simulink model "ControlPendulo2GDL_CICD"  (R2019b)
settings: Solver=ode4  StartTime=0.0  StopTime=ts  FixedStep=0.01  RelTol=1e-3
values from neighbouring files (symbols this model uses):
  b1 = c8    (= 0.01)    [PenduloDatos.m]
  b2 = c8    (= 0.01)    [PenduloDatos.m]
  C = [1 0 0 0]    [PenduloDatos.m]
  g = 9.78    [PenduloDatos.m]
  I1 = 1/12*m1*(a1^2+d1^2)    (= 3.14166666667e-05)    [PenduloDatos.m]
  I2 = 1/12*m2*(a2^2+d2^2)    (= 1.20833333333e-05)    [PenduloDatos.m]
  K = place(Al,Bl,[Pd1 Pd2 Pd3 Pd4])    [PenduloDatos.m]
  K0 = inv(C*(inv(-Al+Bl*K))*Bl)    [PenduloDatos.m]
  L = place(Al',C',[5*Pd1 5*Pd2 5*Pd3 5*Pd4])'    [PenduloDatos.m]
  l1 = c1    (= 0.3)    [PenduloDatos.m]
  l2 = c2    (= 0.2)    [PenduloDatos.m]
  lc1 = 0.25    [PenduloDatos.m]
  lc2 = 0.11    [PenduloDatos.m]
  m1 = c3    (= 0.065)    [PenduloDatos.m]
  m2 = c4    (= 0.025)    [PenduloDatos.m]
  U0 = [Tau1]    [PenduloDatos.m]
  X0 = [Tt1;Tpt1;Tt2;Tpt2]    [PenduloDatos.m]
  XI = [0;0;0;0]    [PenduloDatos.m]
undefined symbols (not defined in the file or in its folder): Al, Bl
libraries: simulink x4
settings Model: Creator=ARQ SEVILLA R  LastModifiedBy=ARQ SEVILLA R

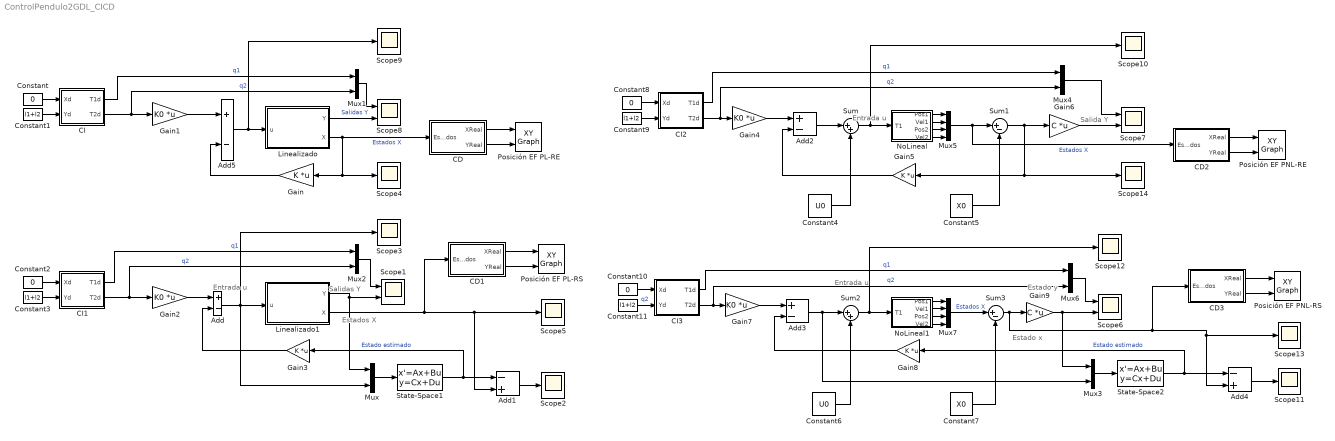
== system ControlPendulo2GDL_CICD ==
  note: Estados X
  note: Salidas Y
  note: Entrada u
  note: Salida Y
  note: Entrada u
  note: Entrada u
  note: Estado y
  note: Estado x
  Add{,2..3,5} (4 alike) : Sum  Inputs=+-
  Add1 : Sum  Inputs=-+
  Add4 : Sum  Inputs=-+
  CD : Subsystem  TreatAsAtomicUnit=on
  CD1 : Subsystem  TreatAsAtomicUnit=on
  CD2 : Subsystem  TreatAsAtomicUnit=on
  CD3 : Subsystem  TreatAsAtomicUnit=on
  CI : Subsystem  TreatAsAtomicUnit=on
  CI1 : Subsystem  TreatAsAtomicUnit=on
  CI2 : Subsystem  TreatAsAtomicUnit=on
  CI3 : Subsystem  TreatAsAtomicUnit=on
  Constant{,2,8,10} (4 alike) : Constant  Value=0
  Constant{1,3,9,11} (4 alike) : Constant  Value=l1+l2
  Constant4 : Constant  Value=U0
  Constant5 : Constant  Value=X0
  Constant6 : Constant  Value=U0
  Constant7 : Constant  Value=X0
  Gain{,3,5,8} (4 alike) : Gain  Gain=K  Multiplication=Matrix(K*u)
  Gain{1..2,4,7} (4 alike) : Gain  Gain=K0  Multiplication=Matrix(K*u)
  Gain6 : Gain  Gain=C  Multiplication=Matrix(K*u)
  Gain9 : Gain  Gain=C  Multiplication=Matrix(K*u)
  Linealizado : Subsystem
  Linealizado1 : Subsystem
  Mux{,1..4,6} (6 alike) : Mux  Inputs=2
  Mux5 : Mux
  Mux7 : Mux
  NoLineal : Subsystem
  NoLineal1 : Subsystem
  Posición EF PL-RE : simulink/Sinks/XY Graph  xmin=-l2-l1  xmax=l2+l1  ymin=-l2-l1  ymax=l2+l1  st=-1
  Posición EF PL-RS : simulink/Sinks/XY Graph  xmin=-l2-l1  xmax=l2+l1  ymin=-l2-l1  ymax=l2+l1  st=-1
  Posición EF PNL-RE : simulink/Sinks/XY Graph  xmin=-l2-l1  xmax=l2+l1  ymin=-l2-l1  ymax=l2+l1  st=-1
  Posición EF PNL-RS : simulink/Sinks/XY Graph  xmin=-l2-l1  xmax=l2+l1  ymin=-l2-l1  ymax=l2+l1  st=-1
  Scope{1,6..8} (4 alike) : Scope  NumInputPorts=2
  Scope{2..5,9..14} (10 alike) : Scope
  State-Space1 : StateSpace  A=Al-L*C  B=[L,Bl]  C=eye(4)  D=zeros(4,2)  InitialCondition=XI
  State-Space2 : StateSpace  A=Al-L*C  B=[L,Bl]  C=eye(4)  D=zeros(4,2)  InitialCondition=XI
  Sum : Sum  Inputs=|++
  Sum1 : Sum  Inputs=|+-
  Sum2 : Sum  Inputs=|++
  Sum3 : Sum  Inputs=|+-
  wires:
  CI/1(T1d) -> Mux1/1  "q1"
  Linealizado/2(X) -> CD/1(Estados), Scope4/1, Gain/1  "Estados X"
  Add5/1 -> Scope9/1, Linealizado/1(u)
  Gain1/1 -> Add5/1
  Linealizado1/2(X) -> CD1/1(Estados), Scope5/1, Add1/2
  Add/1 -> Linealizado1/1(u), Mux/2, Scope3/1
  Gain2/1 -> Add/1
  Linealizado1/1(Y) -> Scope1/2, Mux/1
  Mux/1 -> State-Space1/1
  Add1/1 -> Scope2/1
  Gain3/1 -> Add/2
  State-Space1/1 -> Add1/1, Gain3/1  "Estado estimado"
  CD/1(XReal) -> Posición EF PL-RE/1
  CD/2(YReal) -> Posición EF PL-RE/2
  Constant/1 -> CI/1(Xd)
  Constant1/1 -> CI/2(Yd)
  CI/2(T2d) -> Gain1/1, Mux1/2  "q2"
  Mux1/1 -> Scope8/1
  Linealizado/1(Y) -> Scope8/2  "Salidas Y"
  Gain/1 -> Add5/2
  CD1/2(YReal) -> Posición EF PL-RS/2
  CD1/1(XReal) -> Posición EF PL-RS/1
  Constant2/1 -> CI1/1(Xd)
  Mux2/1 -> Scope1/1
  CI1/1(T1d) -> Mux2/1  "q1"
  Add2/1 -> Sum/1
  Sum/1 -> Scope10/1, NoLineal/1(T1)
  Sum1/1 -> Scope14/1, Gain5/1, Gain6/1
  Sum2/1 -> NoLineal1/1(T1), Scope12/1
  Constant5/1 -> Sum1/2
  Add4/1 -> Scope11/1
  Constant4/1 -> Sum/2
  State-Space2/1 -> Add4/1, Gain8/1  "Estado estimado"
  Constant7/1 -> Sum3/2
  Sum3/1 -> CD3/1(Estados), Scope13/1, Add4/2, Gain9/1
  Add3/1 -> Mux3/2, Sum2/1
  Gain7/1 -> Add3/1
  Gain8/1 -> Add3/2
  Constant6/1 -> Sum2/2
  Gain9/1 -> Mux3/1, Scope6/2
  Gain4/1 -> Add2/1
  Mux3/1 -> State-Space2/1
  Gain5/1 -> Add2/2
  Gain6/1 -> Scope7/2
  Constant8/1 -> CI2/1(Xd)
  CI2/1(T1d) -> Mux4/1  "q1"
  Mux4/1 -> Scope7/1
  NoLineal/3(Pos2) -> Mux5/3
  Mux5/1 -> CD2/1(Estados), Sum1/1  "Estados X"
  NoLineal/4(Vel2) -> Mux5/4
  NoLineal/2(Vel1) -> Mux5/2
  NoLineal/1(Pos1) -> Mux5/1
  CD2/2(YReal) -> Posición EF PNL-RE/2
  CD2/1(XReal) -> Posición EF PNL-RE/1
  Constant10/1 -> CI3/1(Xd)
  Mux6/1 -> Scope6/1
  CI3/1(T1d) -> Mux6/1  "q1"
  CD3/1(XReal) -> Posición EF PNL-RS/1
  CD3/2(YReal) -> Posición EF PNL-RS/2
  NoLineal1/4(Vel2) -> Mux7/4
  NoLineal1/3(Pos2) -> Mux7/3
  NoLineal1/1(Pos1) -> Mux7/1
  NoLineal1/2(Vel1) -> Mux7/2
  Mux7/1 -> Sum3/1  "Estados X"
  Constant3/1 -> CI1/2(Yd)
  CI1/2(T2d) -> Mux2/2, Gain2/1  "q2"
  Constant9/1 -> CI2/2(Yd)
  CI2/2(T2d) -> Mux4/2, Gain4/1  "q2"
  Constant11/1 -> CI3/2(Yd)  "q2"
  CI3/2(T2d) -> Mux6/2, Gain7/1  "q2"

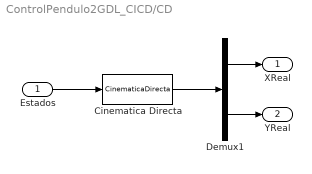
== system ControlPendulo2GDL_CICD/CD ==
  Estados : Inport
  Cinematica Directa : MATLABFcn  MATLABFcn=CinematicaDirecta  OutputDimensions=2
  Demux1 : Demux  Outputs=2
  XReal : Outport  VectorParamsAs1DForOutWhenUnconnected=off
  YReal : Outport  Port=2  VectorParamsAs1DForOutWhenUnconnected=off
  wires:
  Cinematica Directa/1 -> Demux1/1
  Demux1/1 -> XReal/1
  Demux1/2 -> YReal/1
  Estados/1 -> Cinematica Directa/1

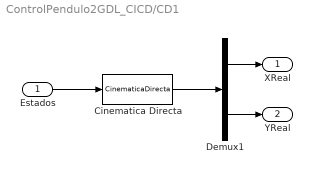
== system ControlPendulo2GDL_CICD/CD1 ==
  Estados : Inport
  Cinematica Directa : MATLABFcn  MATLABFcn=CinematicaDirecta  OutputDimensions=2
  Demux1 : Demux  Outputs=2
  XReal : Outport  VectorParamsAs1DForOutWhenUnconnected=off
  YReal : Outport  Port=2  VectorParamsAs1DForOutWhenUnconnected=off
  wires:
  Estados/1 -> Cinematica Directa/1
  Demux1/2 -> YReal/1
  Demux1/1 -> XReal/1
  Cinematica Directa/1 -> Demux1/1

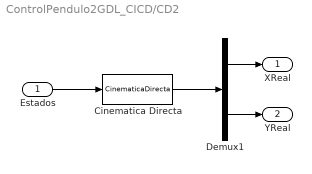
== system ControlPendulo2GDL_CICD/CD2 ==
  Estados : Inport
  Cinematica Directa : MATLABFcn  MATLABFcn=CinematicaDirecta  OutputDimensions=2
  Demux1 : Demux  Outputs=2
  XReal : Outport  VectorParamsAs1DForOutWhenUnconnected=off
  YReal : Outport  Port=2  VectorParamsAs1DForOutWhenUnconnected=off
  wires:
  Cinematica Directa/1 -> Demux1/1
  Demux1/1 -> XReal/1
  Demux1/2 -> YReal/1
  Estados/1 -> Cinematica Directa/1

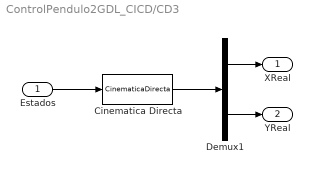
== system ControlPendulo2GDL_CICD/CD3 ==
  Estados : Inport
  Cinematica Directa : MATLABFcn  MATLABFcn=CinematicaDirecta  OutputDimensions=2
  Demux1 : Demux  Outputs=2
  XReal : Outport  VectorParamsAs1DForOutWhenUnconnected=off
  YReal : Outport  Port=2  VectorParamsAs1DForOutWhenUnconnected=off
  wires:
  Estados/1 -> Cinematica Directa/1
  Demux1/2 -> YReal/1
  Demux1/1 -> XReal/1
  Cinematica Directa/1 -> Demux1/1

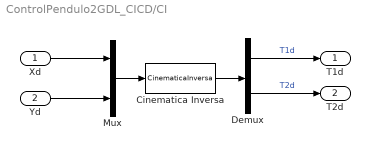
== system ControlPendulo2GDL_CICD/CI ==
  Xd : Inport
  Yd : Inport  Port=2
  Cinematica Inversa : MATLABFcn  MATLABFcn=CinematicaInversa  OutputDimensions=2
  Demux : Demux  Outputs=2
  Mux : Mux  Inputs=2
  T1d : Outport  VectorParamsAs1DForOutWhenUnconnected=off
  T2d : Outport  Port=2  VectorParamsAs1DForOutWhenUnconnected=off
  wires:
  Demux/2 -> T2d/1  "T2d"
  Demux/1 -> T1d/1  "T1d"
  Cinematica Inversa/1 -> Demux/1
  Mux/1 -> Cinematica Inversa/1
  Xd/1 -> Mux/1
  Yd/1 -> Mux/2

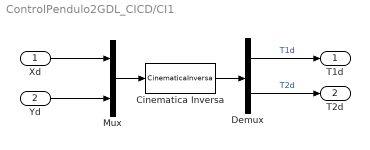
== system ControlPendulo2GDL_CICD/CI1 ==
  Xd : Inport
  Yd : Inport  Port=2
  Cinematica Inversa : MATLABFcn  MATLABFcn=CinematicaInversa  OutputDimensions=2
  Demux : Demux  Outputs=2
  Mux : Mux  Inputs=2
  T1d : Outport  VectorParamsAs1DForOutWhenUnconnected=off
  T2d : Outport  Port=2  VectorParamsAs1DForOutWhenUnconnected=off
  wires:
  Yd/1 -> Mux/2
  Xd/1 -> Mux/1
  Mux/1 -> Cinematica Inversa/1
  Cinematica Inversa/1 -> Demux/1
  Demux/1 -> T1d/1  "T1d"
  Demux/2 -> T2d/1  "T2d"

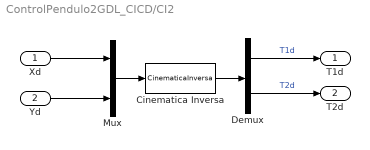
== system ControlPendulo2GDL_CICD/CI2 ==
  Xd : Inport
  Yd : Inport  Port=2
  Cinematica Inversa : MATLABFcn  MATLABFcn=CinematicaInversa  OutputDimensions=2
  Demux : Demux  Outputs=2
  Mux : Mux  Inputs=2
  T1d : Outport  VectorParamsAs1DForOutWhenUnconnected=off
  T2d : Outport  Port=2  VectorParamsAs1DForOutWhenUnconnected=off
  wires:
  Demux/2 -> T2d/1  "T2d"
  Demux/1 -> T1d/1  "T1d"
  Cinematica Inversa/1 -> Demux/1
  Mux/1 -> Cinematica Inversa/1
  Xd/1 -> Mux/1
  Yd/1 -> Mux/2

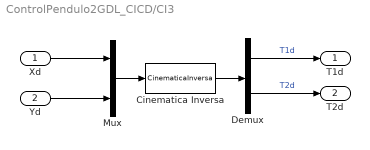
== system ControlPendulo2GDL_CICD/CI3 ==
  Xd : Inport
  Yd : Inport  Port=2
  Cinematica Inversa : MATLABFcn  MATLABFcn=CinematicaInversa  OutputDimensions=2
  Demux : Demux  Outputs=2
  Mux : Mux  Inputs=2
  T1d : Outport  VectorParamsAs1DForOutWhenUnconnected=off
  T2d : Outport  Port=2  VectorParamsAs1DForOutWhenUnconnected=off
  wires:
  Yd/1 -> Mux/2
  Xd/1 -> Mux/1
  Mux/1 -> Cinematica Inversa/1
  Cinematica Inversa/1 -> Demux/1
  Demux/1 -> T1d/1  "T1d"
  Demux/2 -> T2d/1  "T2d"

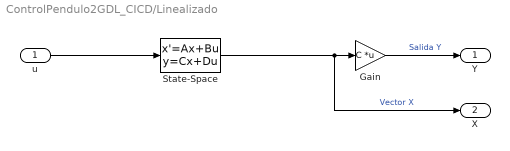
== system ControlPendulo2GDL_CICD/Linealizado ==
  u : Inport
  Gain : Gain  Gain=C  Multiplication=Matrix(K*u)
  State-Space : StateSpace  A=Al  B=Bl  C=eye(4)  D=zeros(4,1)  InitialCondition=XI
  Y : Outport
  X : Outport  Port=2
  wires:
  State-Space/1 -> X/1, Gain/1  "Vector X"
  Gain/1 -> Y/1  "Salida Y"
  u/1 -> State-Space/1

== system ControlPendulo2GDL_CICD/Linealizado1 ==
  u : Inport
  Gain : Gain  Gain=C  Multiplication=Matrix(K*u)
  State-Space : StateSpace  A=Al  B=Bl  C=eye(4)  D=zeros(4,1)  InitialCondition=XI
  Y : Outport
  X : Outport  Port=2
  wires:
  u/1 -> State-Space/1
  Gain/1 -> Y/1  "Salida Y"
  State-Space/1 -> Gain/1, X/1  "Vector X"

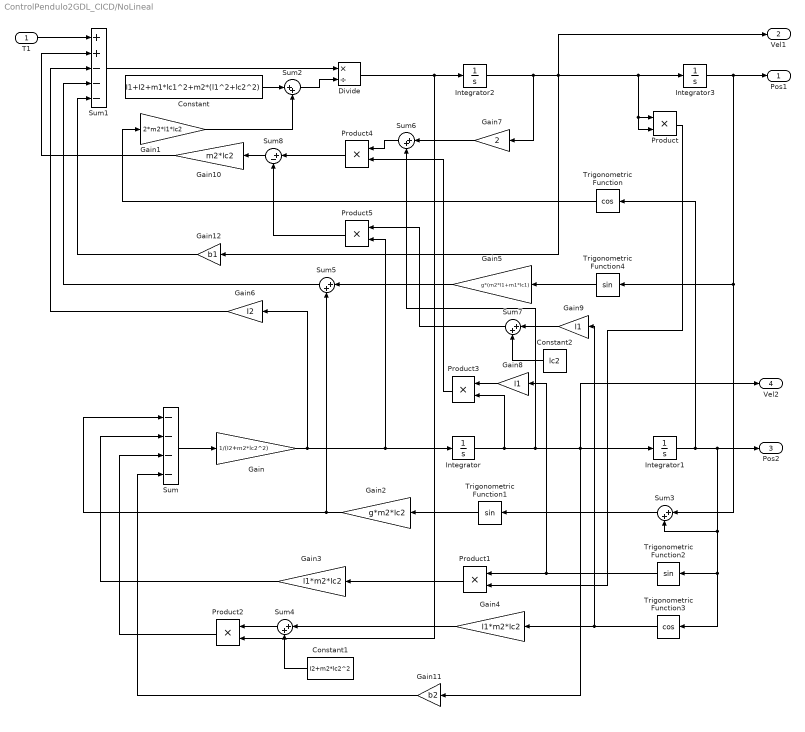
== system ControlPendulo2GDL_CICD/NoLineal ==
  T1 : Inport
  Constant : Constant  Value=I1+I2+m1*lc1^2+m2*(l1^2+lc2^2)
  Constant1 : Constant  Value=I2+m2*lc2^2
  Constant2 : Constant  Value=lc2
  Divide : Product  Inputs=*/
  Gain : Gain  Gain=1/(I2+m2*lc2^2)
  Gain1 : Gain  Gain=2*m2*l1*lc2
  Gain10 : Gain  Gain=m2*lc2
  Gain11 : Gain  Gain=b2
  Gain12 : Gain  Gain=b1
  Gain2 : Gain  Gain=g*m2*lc2
  Gain3 : Gain  Gain=l1*m2*lc2
  Gain4 : Gain  Gain=l1*m2*lc2
  Gain5 : Gain  Gain=g*(m2*l1+m1*lc1)
  Gain6 : Gain  Gain=I2
  Gain7 : Gain  Gain=2
  Gain8 : Gain  Gain=l1
  Gain9 : Gain  Gain=l1
  Integrator : Integrator  InitialCondition=XI(4)
  Integrator1 : Integrator  InitialCondition=XI(3)
  Integrator2 : Integrator  InitialCondition=XI(2)
  Integrator3 : Integrator  InitialCondition=XI(1)
  Product{,1..5} (6 alike) : Product
  Sum : Sum  Inputs=----
  Sum1 : Sum  Inputs=++---
  Sum{2..7} (6 alike) : Sum  Inputs=|++
  Sum8 : Sum  Inputs=|+-
  Trigonometric Function : Trigonometry  Operator=cos
  Trigonometric Function1 : Trigonometry
  Trigonometric Function2 : Trigonometry
  Trigonometric Function3 : Trigonometry  Operator=cos
  Trigonometric Function4 : Trigonometry
  Pos1 : Outport  VectorParamsAs1DForOutWhenUnconnected=off
  Vel1 : Outport  Port=2  VectorParamsAs1DForOutWhenUnconnected=off
  Pos2 : Outport  Port=3  VectorParamsAs1DForOutWhenUnconnected=off
  Vel2 : Outport  Port=4  VectorParamsAs1DForOutWhenUnconnected=off
  wires:
  Integrator/1 -> Product3/2, Vel2/1, Integrator1/1, Gain11/1, Sum6/2
  Product4/1 -> Sum8/1
  Gain10/1 -> Sum1/2
  Constant/1 -> Sum2/1
  Sum7/1 -> Product5/1
  Sum1/1 -> Divide/1
  Gain6/1 -> Sum1/3
  Integrator1/1 -> Trigonometric Function/1, Trigonometric Function3/1, Trigonometric Function2/1, Sum3/2, Pos2/1
  Sum3/1 -> Trigonometric Function1/1
  Gain11/1 -> Sum/4
  Product/1 -> Product1/2
  Gain4/1 -> Sum4/1
  Sum/1 -> Gain/1
  Constant2/1 -> Sum7/2
  Gain8/1 -> Product3/1
  Trigonometric Function3/1 -> Gain9/1, Gain4/1
  Product1/1 -> Gain3/1
  Gain7/1 -> Sum6/1
  Trigonometric Function2/1 -> Gain8/1, Product1/1
  Sum8/1 -> Gain10/1
  Gain2/1 -> Sum5/2, Sum/1
  Constant1/1 -> Sum4/2
  Integrator2/1 -> Gain7/1, Vel1/1, Gain12/1, Product/2, Product/1, Integrator3/1
  Trigonometric Function4/1 -> Gain5/1
  Divide/1 -> Product2/2, Integrator2/1
  Product5/1 -> Sum8/2
  Gain3/1 -> Sum/2
  Gain9/1 -> Sum7/1
  T1/1 -> Sum1/1
  Gain/1 -> Product5/2, Integrator/1, Gain6/1
  Product3/1 -> Product4/2
  Sum2/1 -> Divide/2
  Sum6/1 -> Product4/1
  Integrator3/1 -> Pos1/1, Sum3/1, Trigonometric Function4/1
  Trigonometric Function/1 -> Gain1/1
  Gain1/1 -> Sum2/2
  Sum5/1 -> Sum1/4
  Gain5/1 -> Sum5/1
  Gain12/1 -> Sum1/5
  Product2/1 -> Sum/3
  Sum4/1 -> Product2/1
  Trigonometric Function1/1 -> Gain2/1

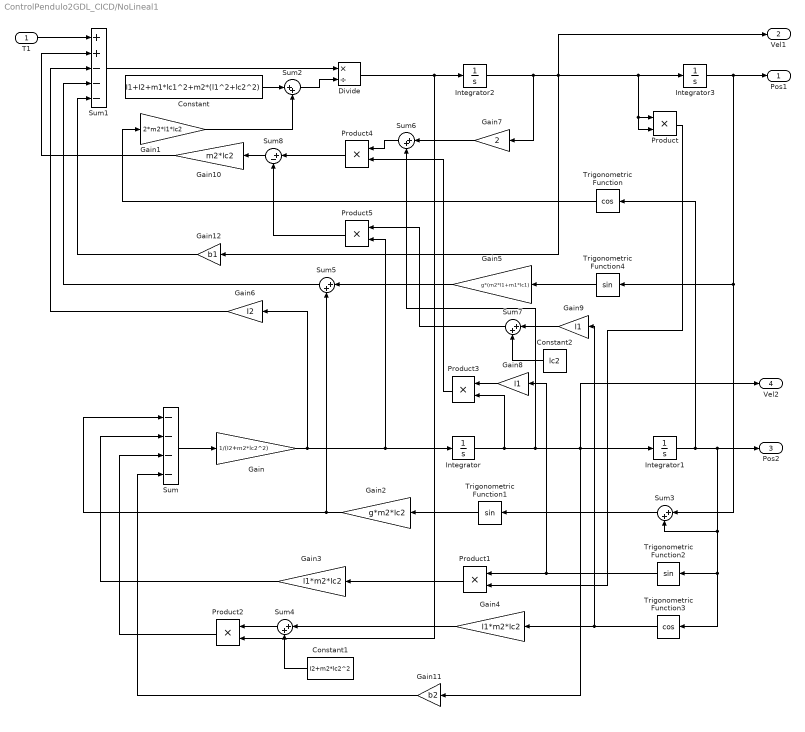
== system ControlPendulo2GDL_CICD/NoLineal1 ==
  T1 : Inport
  Constant : Constant  Value=I1+I2+m1*lc1^2+m2*(l1^2+lc2^2)
  Constant1 : Constant  Value=I2+m2*lc2^2
  Constant2 : Constant  Value=lc2
  Divide : Product  Inputs=*/
  Gain : Gain  Gain=1/(I2+m2*lc2^2)
  Gain1 : Gain  Gain=2*m2*l1*lc2
  Gain10 : Gain  Gain=m2*lc2
  Gain11 : Gain  Gain=b2
  Gain12 : Gain  Gain=b1
  Gain2 : Gain  Gain=g*m2*lc2
  Gain3 : Gain  Gain=l1*m2*lc2
  Gain4 : Gain  Gain=l1*m2*lc2
  Gain5 : Gain  Gain=g*(m2*l1+m1*lc1)
  Gain6 : Gain  Gain=I2
  Gain7 : Gain  Gain=2
  Gain8 : Gain  Gain=l1
  Gain9 : Gain  Gain=l1
  Integrator : Integrator  InitialCondition=XI(4)
  Integrator1 : Integrator  InitialCondition=XI(3)
  Integrator2 : Integrator  InitialCondition=XI(2)
  Integrator3 : Integrator  InitialCondition=XI(1)
  Product{,1..5} (6 alike) : Product
  Sum : Sum  Inputs=----
  Sum1 : Sum  Inputs=++---
  Sum{2..7} (6 alike) : Sum  Inputs=|++
  Sum8 : Sum  Inputs=|+-
  Trigonometric Function : Trigonometry  Operator=cos
  Trigonometric Function1 : Trigonometry
  Trigonometric Function2 : Trigonometry
  Trigonometric Function3 : Trigonometry  Operator=cos
  Trigonometric Function4 : Trigonometry
  Pos1 : Outport  VectorParamsAs1DForOutWhenUnconnected=off
  Vel1 : Outport  Port=2  VectorParamsAs1DForOutWhenUnconnected=off
  Pos2 : Outport  Port=3  VectorParamsAs1DForOutWhenUnconnected=off
  Vel2 : Outport  Port=4  VectorParamsAs1DForOutWhenUnconnected=off
  wires:
  Integrator/1 -> Product3/2, Vel2/1, Integrator1/1, Gain11/1, Sum6/2
  Product4/1 -> Sum8/1
  Gain10/1 -> Sum1/2
  Constant/1 -> Sum2/1
  Sum7/1 -> Product5/1
  Sum1/1 -> Divide/1
  Gain6/1 -> Sum1/3
  Integrator1/1 -> Trigonometric Function/1, Trigonometric Function3/1, Trigonometric Function2/1, Sum3/2, Pos2/1
  Sum3/1 -> Trigonometric Function1/1
  Gain11/1 -> Sum/4
  Product/1 -> Product1/2
  Gain4/1 -> Sum4/1
  Sum/1 -> Gain/1
  Constant2/1 -> Sum7/2
  Gain8/1 -> Product3/1
  Trigonometric Function3/1 -> Gain9/1, Gain4/1
  Product1/1 -> Gain3/1
  Gain7/1 -> Sum6/1
  Trigonometric Function2/1 -> Gain8/1, Product1/1
  Sum8/1 -> Gain10/1
  Gain2/1 -> Sum5/2, Sum/1
  Constant1/1 -> Sum4/2
  Integrator2/1 -> Gain7/1, Vel1/1, Gain12/1, Product/2, Product/1, Integrator3/1
  Trigonometric Function4/1 -> Gain5/1
  Divide/1 -> Product2/2, Integrator2/1
  Product5/1 -> Sum8/2
  Gain3/1 -> Sum/2
  Gain9/1 -> Sum7/1
  T1/1 -> Sum1/1
  Gain/1 -> Product5/2, Integrator/1, Gain6/1
  Product3/1 -> Product4/2
  Sum2/1 -> Divide/2
  Sum6/1 -> Product4/1
  Integrator3/1 -> Pos1/1, Sum3/1, Trigonometric Function4/1
  Trigonometric Function/1 -> Gain1/1
  Gain1/1 -> Sum2/2
  Sum5/1 -> Sum1/4
  Gain5/1 -> Sum5/1
  Gain12/1 -> Sum1/5
  Product2/1 -> Sum/3
  Sum4/1 -> Product2/1
  Trigonometric Function1/1 -> Gain2/1
